simulink model "lateral_autopilot_full"  (R2016b)
settings: Solver=VariableStepAuto  StartTime=0.0  StopTime=t_end  RelTol=1e-3
values from neighbouring files (symbols this model uses):
  A = [- 0.322 -1.12 ... (first row only)    [dutch_roll_mode_2_1.m]    (also in parameters_longitudal_autopilot.m = [ -0.322 0.052 0.028 -1.12 0.002)
  B = [0;0]    [dutch_roll_mode_2_1.m]    (also in parameters_longitudal_autopilot.m = [ 0 0 0 0 10]')
  C = [0 0 0 1 0 ... (first row only)    [parameters_longitudal_autopilot.m]
  chi_c = 10*deg2rad    [run_task_2f.m]
  D = [0 0 0 0]'    [parameters_longitudal_autopilot.m]
  delta_a_max = 25*deg2rad    (= 0.436332312999)    [parameters_longitudal_autopilot.m]    (also in regulation_parameters_2_2.m = 1432.39448783)
  g = 9.81    [parameters_longitudal_autopilot.m]
  k_d_phi = (2*zeta_phi*omega_n_phi - a_phi_1) / a_phi_2    [parameters_longitudal_autopilot.m]    (also in regulation_parameters_2_2.m)
  k_i_chi = omega_n_chi^2*V_g/g    [parameters_longitudal_autopilot.m]
  k_i_phi = 0    [parameters_longitudal_autopilot.m]
  k_p_chi = 2*zeta_chi*omega_n_chi*V_g/g    [parameters_longitudal_autopilot.m]
  k_p_phi = sign(a_phi_2)*delta_a_max /e_phi_max    [parameters_longitudal_autopilot.m]    (also in regulation_parameters_2_2.m = 1.66666666667)
  V_g = 637/3.6    (= 176.944444444)    [parameters_longitudal_autopilot.m]    (also in regulation_parameters_2_2.m = 2293.2)
settings Model: Creator=EllaLovise  LastModifiedBy=Alexandra

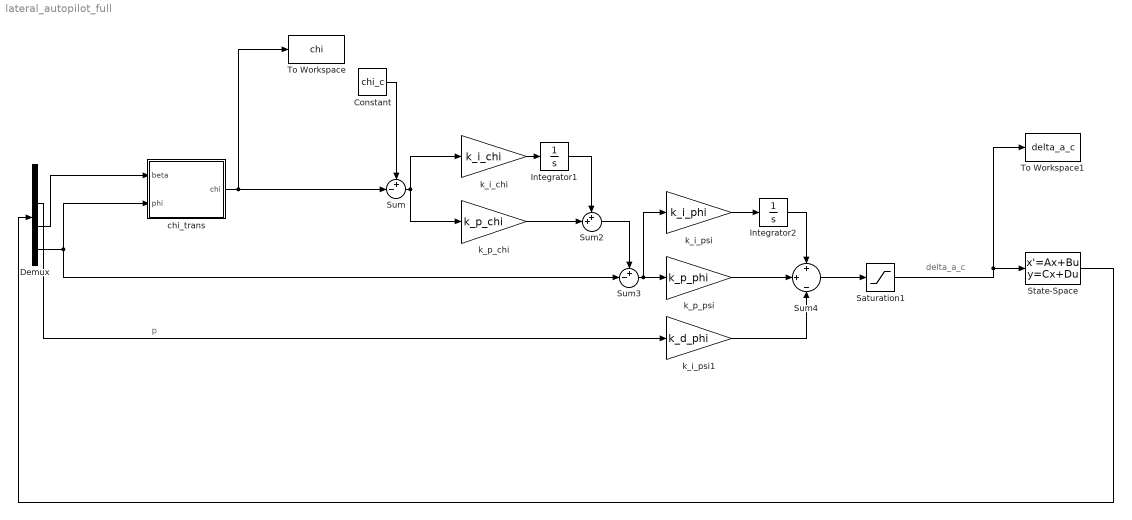
== system lateral_autopilot_full ==
  note: delta_a_c
  note: p
  Constant : Constant  Value=chi_c
  Demux : Demux
  Integrator1 : Integrator
  Integrator2 : Integrator
  Saturation1 : Saturate  UpperLimit=delta_a_max  LowerLimit=-1*delta_a_max
  State-Space : StateSpace  A=A  B=B  C=C  D=D  X0=0
  Sum : Sum  Inputs=+-|
  Sum2 : Sum  Inputs=++|
  Sum3 : Sum  Inputs=+-|
  Sum4 : Sum  Inputs=+|+|-
  To Workspace : ToWorkspace  VariableName=chi  SaveFormat=Structure With Time  SampleTime=-1
  To Workspace1 : ToWorkspace  VariableName=delta_a_c  SaveFormat=Structure With Time  SampleTime=-1
  chi_trans : Subsystem
  k_i_chi : Gain  Gain=k_i_chi
  k_i_psi : Gain  Gain=k_i_phi
  k_i_psi1 : Gain  Gain=k_d_phi
  k_p_chi : Gain  Gain=k_p_chi
  k_p_psi : Gain  Gain=k_p_phi
  wires:
  Constant/1 -> Sum/1
  State-Space/1 -> Demux/1
  Sum/1 -> k_i_chi/1, k_p_chi/1
  k_p_chi/1 -> Sum2/2
  Sum2/1 -> Sum3/1
  Sum3/1 -> k_i_psi/1, k_p_psi/1
  k_i_psi/1 -> Integrator2/1
  chi_trans/1(chi) -> Sum/2, To Workspace/1
  k_i_chi/1 -> Integrator1/1
  Integrator1/1 -> Sum2/1
  Integrator2/1 -> Sum4/1
  k_p_psi/1 -> Sum4/2
  k_i_psi1/1 -> Sum4/3
  Demux/4 -> Sum3/2, chi_trans/2(phi)
  Demux/3 -> chi_trans/1(beta)
  Demux/2 -> k_i_psi1/1
  Saturation1/1 -> To Workspace1/1, State-Space/1
  Sum4/1 -> Saturation1/1

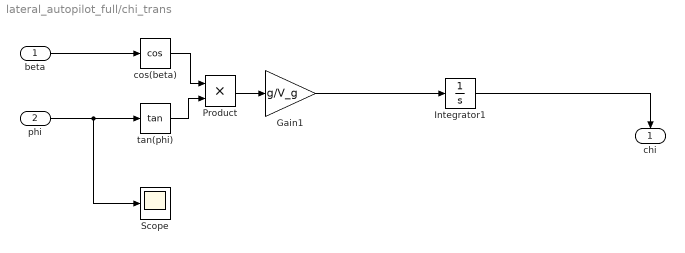
== system lateral_autopilot_full/chi_trans ==
  beta : Inport
  phi : Inport  Port=2
  Gain1 : Gain  Gain=g/V_g
  Integrator1 : Integrator
  Product : Product
  Scope : Scope
  cos(beta) : Trigonometry  Operator=cos
  tan(phi) : Trigonometry  Operator=tan
  chi : Outport
  wires:
  phi/1 -> Scope/1, tan(phi)/1
  Integrator1/1 -> chi/1
  beta/1 -> cos(beta)/1
  tan(phi)/1 -> Product/2
  Product/1 -> Gain1/1
  cos(beta)/1 -> Product/1
  Gain1/1 -> Integrator1/1
